simulink model "KF_test"  (R2016b)
settings: Solver=VariableStepAuto  StartTime=0.0  StopTime=10.0  RelTol=1e-3
values from neighbouring files (symbols this model uses):
  H = diag([1 1])    [init_KF_test.m]
undefined symbols (not defined in the file or in its folder): DELTA, GAMMA, PHI
settings Model: Creator=helene  LastModifiedBy=helene

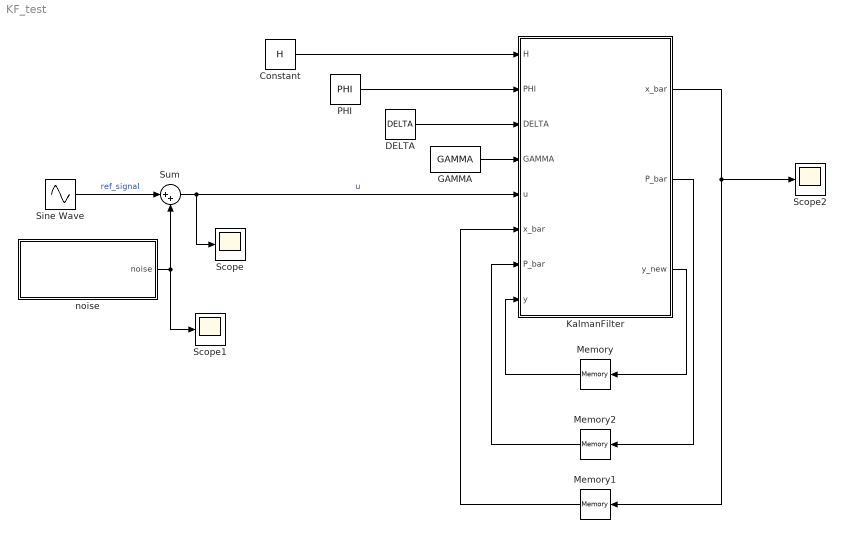
== system KF_test ==
  Constant : Constant  Value=H
  DELTA : Constant  Value=DELTA
  GAMMA : Constant  Value=GAMMA
  KalmanFilter : MATLAB Function  TreatAsAtomicUnit=on
  Memory : Memory  X0=[0 0 ]
  Memory1 : Memory  X0=[0 0]'
  Memory2 : Memory  X0=[0 0; 0 0]
  PHI : Constant  Value=PHI
  Scope : Scope
  Scope1 : Scope
  Scope2 : Scope
  Sine Wave : Sin  SampleTime=0
  Sum : Sum  Inputs=|++
  noise : MATLAB Function  TreatAsAtomicUnit=on
  wires:
  PHI/1 -> KalmanFilter/2(PHI)
  GAMMA/1 -> KalmanFilter/4(GAMMA)
  DELTA/1 -> KalmanFilter/3(DELTA)
  Sum/1 -> KalmanFilter/5(u), Scope/1  "u"
  Sine Wave/1 -> Sum/1  "ref_signal"
  noise/1(noise) -> Scope1/1, Sum/2
  KalmanFilter/3(y_new) -> Memory/1
  Memory/1 -> KalmanFilter/8(y)
  Constant/1 -> KalmanFilter/1(H)
  KalmanFilter/1(x_bar) -> Scope2/1, Memory1/1
  Memory1/1 -> KalmanFilter/6("x_bar ")
  KalmanFilter/2(P_bar) -> Memory2/1
  Memory2/1 -> KalmanFilter/7("P_bar ")

== matlab function KF_test/noise ==
  data: noise output
function  noise = NoiseGenerator()

deg2rad = pi/180;

var = (15*deg2rad)^2;
noise = sqrt(var)*randn()

== matlab function KF_test/KalmanFilter ==
  data: x_bar output; P_bar output; H input; PHI input; DELTA input; GAMMA input; u input; x_bar input; P_bar input; y_new output; y input
function [x_bar,P_bar,y_new]= KalmanFilter(H, PHI,DELTA,GAMMA,u, x_bar,P_bar,y)

% 2) Defining Q and R
Q = diag([1 1]); 
R = diag([1 1]);

% 3) Calculate optimal Kalman gain K
K = P_bar*H'*(H*P_bar*H' + R)^-1;

% 4) Update state estimate x_hat
x_hat = x_bar + K*(y - H*x_bar);

% 5) Update co.var.m P_hat
P_hat = (eye(2) - K*H)*P_bar*(eye(2)-K*H)' + K*R*K';

% 6) Update x_bar
x_bar = PHI*x_hat + DELTA*u;

% 7) Update covariance matrix P

P_bar = PHI*P_hat*PHI' + GAMMA'*Q*GAMMA;

% P_ = PHI*P_hat*PHI' + GAMMA*Q*GAMMA';

y_new = Q*y;
